simulink library "pathProjectionNumerical_ul"  (R2018b)
settings: Solver=VariableStepAuto  StartTime=0.0  StopTime=10.0  RelTol=1e-3
undefined symbols (not defined in the file or in its folder): searchDistance_none
settings Model: Creator=mcobb  LastModifiedBy=mitch
settings DebuggingCC: LibraryContextMissingDiagnostic=none
settings SFSimCC: SimUseLocalCustomCode=off
settings RTWCC: RTWUseLocalCustomCode=off

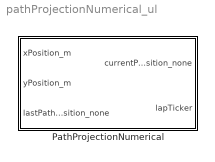
== system pathProjectionNumerical_ul ==
  PathProjectionNumerical : Subsystem  mask{sDist=searchDistance_none, brkpts=linspace(0,1), xVals=sin(linspace(0,1)), yVals=sin(linspace(0,1))}
      mask prompts: sDist "Search Distance"; brkpts "Breakpoints"; xVals "X Values"; yVals "Y Values"
      mask init:
      | pathProjectionNumerical_init

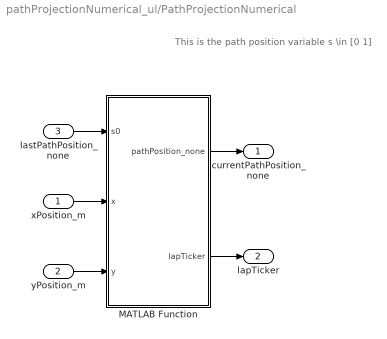
== system pathProjectionNumerical_ul/PathProjectionNumerical ==
  note: This is the path position variable s \in [0 1]
  xPosition_m : Inport
  yPosition_m : Inport  Port=2
  lastPathPosition_none : Inport  Port=3
  MATLAB Function : MATLAB Function  TreatAsAtomicUnit=on
  currentPathPosition_none : Outport  PortDimensions=1
  lapTicker : Outport  Port=2  PortDimensions=1
  wires:
  xPosition_m/1 -> MATLAB Function/2(x)
  yPosition_m/1 -> MATLAB Function/3(y)
  MATLAB Function/1(pathPosition_none) -> currentPathPosition_none/1
  lastPathPosition_none/1 -> MATLAB Function/1(s0)
  MATLAB Function/2(lapTicker) -> lapTicker/1

== matlab function pathProjectionNumerical_ul/PathProjectionNumerical/MATLAB Function ==
  data: s0 input; pathPosition_none output; x input; y input; lapTicker output; brkpts parameter; xVals parameter; yVals parameter; sDist parameter
function [pathPosition_none,lapTicker] = fcn(s0,x,y,...
    brkpts, xVals, yVals, sDist)
pathPosition_none=0;
lapTicker=0;
coder.extrinsic('pathProjectionNumerical')

[pathPosition_none,lapTicker] = pathProjectionNumerical(s0,x,y,brkpts, xVals, yVals, sDist);

end
